simulink model "gate_V22_2016a"  (R2016b)
settings: Solver=FixedStepAuto  StartTime=0.0  StopTime=100  FixedStep=0.001  RelTol=1e-3  EnableMultiTasking=on
values from neighbouring files (symbols this model uses):
  CLOSE_CHAR = CHAR_STAR    (= 42)    [GateParameter.m]
  CLOSE_SIDE_VALUE = 2.95*oneSec    (= 2950)    [GateParameter.m]
  CLOSED = 12    [GateParameter.m]
  CLOSING = 13    [GateParameter.m]
  NO_PASS_ASSIG = 6    [GateParameter.m]
  OPEN = 14    [GateParameter.m]
  OPEN_CHAR = CHAR_HASH    (= 35)    [GateParameter.m]
  OPEN_SIDE_VALUE = 3*oneSec    (= 3000)    [GateParameter.m]
  OPEN_TIMEOUT = 60*oneSec    (= 60000)    [GateParameter.m]
  OPENING = 11    [GateParameter.m]
  OPENING_ACTIVE = 1    [GateParameter.m]
  PASS_ASSIGNED = 7    [GateParameter.m]
  PASS_INCOMPLETE = 8    [GateParameter.m]
  PASS_TIMEOUT = 10*oneSec    (= 10000)    [GateParameter.m]
  PASSWORD_VERIFIED = 5    [GateParameter.m]
  TIMEOUT = 9    [GateParameter.m]
  WRONG_PASSWORD = 2    [GateParameter.m]
undefined symbols (not defined in the file or in its folder): sigbuilder_block
libraries: simulink x9, arduinolib x4
(part 3 of 3)

== stateflow chart gate_V22_2016a/HardwareOutputWrapper/C_HardwareOutputWrapper_RF/MotorHandler/MotorsHandler ==
  state MonitorChange
  state UpdatePins
    (default) -> (junction 91) : /* updating motor Pins Switch case */
    (junction 91) -> (junction 92) [order 1] : [(leftMotor == OPENING) && ((rightMotor == CLOSED) || (rightMotor == OPEN))]
    (junction 92) -> (junction 100) : {LeftPin = true;...
        | ComPin = true;...
        | RightPin = false;}
    (junction 91) -> (junction 93) [order 2]
    (junction 93) -> (junction 94) [order 1] : [(leftMotor == CLOSING) && ((rightMotor == CLOSED) || (rightMotor == OPEN))]
    (junction 94) -> (junction 99) : {LeftPin = false;...
        | ComPin = false;...
        |  RightPin = true;}
    (junction 93) -> (junction 95) [order 2]
    (junction 95) -> (junction 96) [order 1] : [(rightMotor == CLOSING) && ((leftMotor == CLOSED) || (leftMotor == OPEN))]
    (junction 96) -> (junction 98) : {LeftPin = true;...
        | ComPin = false;...
        | RightPin = false;}
    (junction 95) -> (junction 102) [order 2]
    (junction 102) -> (junction 103) [order 1] : [(rightMotor == OPENING) && ((leftMotor == CLOSED) || (leftMotor == OPEN))]
    (junction 103) -> (junction 110) : {LeftPin = false;...
        | ComPin = true;...
        | RightPin = true;}
    (junction 102) -> (junction 104) [order 2]
    (junction 104) -> (junction 105) [order 1] : [(rightMotor == OPENING) && (leftMotor == OPENING)]
    (junction 105) -> (junction 111) : {LeftPin = true;...
        | ComPin = true;...
        | RightPin = true;}
    (junction 104) -> (junction 106) [order 2]
    (junction 106) -> (junction 107) [order 1] : [(rightMotor == CLOSING) && (leftMotor == CLOSING)]
    (junction 107) -> (junction 112) : {LeftPin = false;...
        | ComPin = false;...
        | RightPin = false;}
    (junction 106) -> (junction 123) [order 2]
    (junction 123) -> (junction 124) [order 1] : [((rightMotor == CLOSED) || (rightMotor == OPEN)) ...
        | && ((leftMotor == CLOSED) || (leftMotor == OPEN))]
    (junction 123) -> (junction 97) [order 2]
    (junction 124) -> (junction 125) : {LeftPin = false;...
        | ComPin = true;...
        | RightPin = false;}
    (junction 100) -> (junction 99)
    (junction 99) -> (junction 98)
    (junction 98) -> (junction 110)
    (junction 125) -> (junction 97)
    (junction 112) -> (junction 125)
    (junction 111) -> (junction 112)
    (junction 110) -> (junction 111)
    (junction 97) -> (junction 101)
  (default) -> MonitorChange
  UpdatePins -> MonitorChange
  MonitorChange -> UpdatePins : [(leftMotor != oldLeft) ...
      | || (rightMotor != oldRight)]
  data: LeftPin output =false; ComPin output =true; RightPin output =false; leftMotor input; oldLeft input; rightMotor input; oldRight input; CLOSED input; CLOSING input; OPEN input; OPENING input

== stateflow chart gate_V22_2016a/HardwareInputWrapper/MIL/CurrentFilterSubsystem/10msSmapler ==
  (default) -> (junction 2)
  (junction 2) -> (junction 3) : {counter_1ms++;}
  (junction 3) -> (junction 6) : [counter_1ms == 10]
      | {
      | triggerOn;
      | counter_1ms = 0;
      | }
  data: counter_1ms local double
  events: triggerOn output FUNCTION_CALL_EVENT
